simulink model "agriculture"  (R2016a)
settings: Solver=VariableStepAuto  StartTime=0.0  StopTime=10.0  RelTol=1e-3
libraries: simulink x1
settings Model: Creator=desilvtk  LastModifiedBy=desilvtk

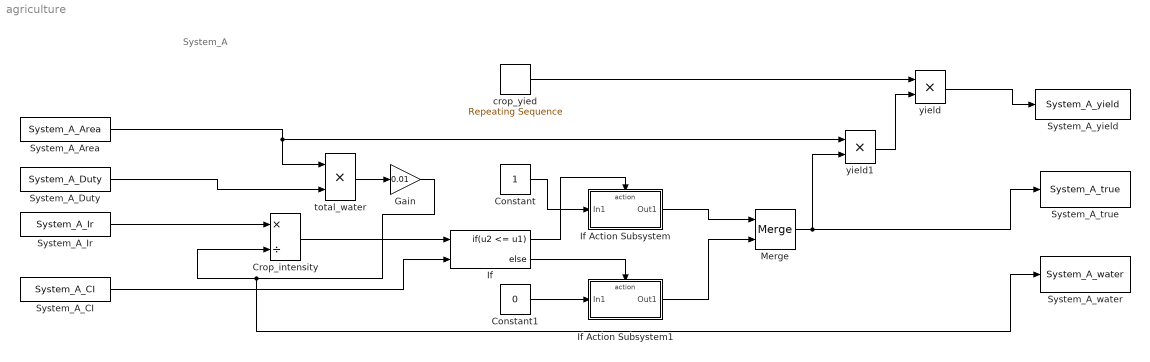
== system agriculture ==
  note: System_A
  Constant : Constant
  Constant1 : Constant  Value=0
  Crop_intensity : Product  Inputs=*/
  Gain : Gain  Gain=0.01
  If : If  NumInputs=2  IfExpression=u2 <= u1
  If Action Subsystem : Subsystem  TreatAsAtomicUnit=on
  If Action Subsystem1 : Subsystem  TreatAsAtomicUnit=on
  Merge : Merge
  System_A_Area : FromWorkspace  VariableName=System_A_Area  SampleTime=0
  System_A_CI : FromWorkspace  VariableName=System_A_CI  SampleTime=0
  System_A_Duty : FromWorkspace  VariableName=System_A_Duty  SampleTime=0
  System_A_Ir : FromWorkspace  VariableName=System_A_Ir  SampleTime=0
  System_A_true : ToWorkspace  VariableName=System_A_true  SaveFormat=Timeseries  SampleTime=-1
  System_A_water : ToWorkspace  VariableName=System_A_water  SaveFormat=Timeseries  SampleTime=-1
  System_A_yield : ToWorkspace  VariableName=System_A_yield  SaveFormat=Timeseries  SampleTime=-1
  crop_yied : simulink/Sources/Repeating Sequence  rep_seq_t=[1,2,3,4,5,6,7,8,9,10,11,12]  rep_seq_y=[5.3,5.3,5.3,5.3,5.3,5.3,5.4,5.4,5.4,5.4,5.4,5.4]
  total_water : Product  Inputs=**
  yield : Product
  yield1 : Product
  wires:
  yield/1 -> System_A_yield/1
  Merge/1 -> System_A_true/1, yield1/2
  Gain/1 -> Crop_intensity/2, System_A_water/1
  yield1/1 -> yield/2
  crop_yied/1 -> yield/1
  If Action Subsystem1/1(Out1) -> Merge/2
  If Action Subsystem/1(Out1) -> Merge/1
  total_water/1 -> Gain/1
  System_A_CI/1 -> If/2
  Constant1/1 -> If Action Subsystem1/1(In1)
  Constant/1 -> If Action Subsystem/1(In1)
  If/2 -> If Action Subsystem1/Action
  If/1 -> If Action Subsystem/Action
  Crop_intensity/1 -> If/1
  System_A_Duty/1 -> total_water/2
  System_A_Ir/1 -> Crop_intensity/1
  System_A_Area/1 -> total_water/1, yield1/1

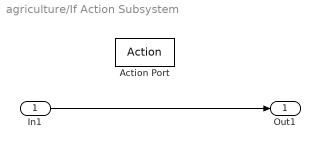
== system agriculture/If Action Subsystem ==
  In1 : Inport
  Action Port : ActionPort  ActionType=then
  Out1 : Outport
  wires:
  In1/1 -> Out1/1

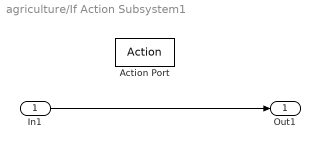
== system agriculture/If Action Subsystem1 ==
  In1 : Inport
  Action Port : ActionPort  ActionType=else
  Out1 : Outport
  wires:
  In1/1 -> Out1/1
